simulink model "blockdemo"  (Simulink 6.3)
settings: Solver=FixedStepDiscrete  StartTime=0.0  StopTime=20  FixedStep=1  RelTol=1e-3
InitFcn:
  | %% DSPBuilder Start
  | alt_dspbuilder_update_model(bdroot)
  | %% DSPBuilder End
libraries: allblocks_alteradspbuilder2 x5
settings Model: Creator=cpurcell  LastModifiedBy=delphick
settings OptimizationCC: BlockReduction=off  BooleanDataType=off  InlineInvariantSignals=on
settings DebuggingCC: SolverPrmCheckMsg=none
settings HardwareCC: TargetUnknown=on

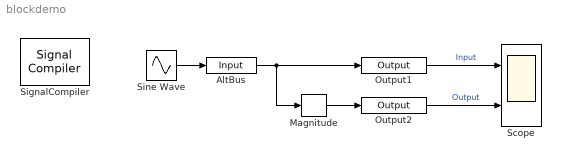
== system blockdemo ==
  AltBus : allblocks_alteradspbuilder2/Input  iofile=C:\workspace_clean\Documentation\DesignExamples\Tutorials\UnitBlocks\Arithmetic\Magnitude\tb_blockdemo\blockdemo_AltBus.salt  BusType=Signed Integer  bwl=5  bwr=4  SpecifyClock=off  PORTTYPE=Input
  Magnitude : allblocks_alteradspbuilder2/Magnitude
  Output1 : allblocks_alteradspbuilder2/Output  iofile=C:\workspace_clean\Documentation\DesignExamples\Tutorials\UnitBlocks\Arithmetic\Magnitude\tb_blockdemo\blockdemo_Output1.capture  BusType=Signed Integer  bwl=5  bwr=0  PORTTYPE=Output
  Output2 : allblocks_alteradspbuilder2/Output  iofile=C:\workspace_clean\Documentation\DesignExamples\Tutorials\UnitBlocks\Arithmetic\Magnitude\tb_blockdemo\blockdemo_Output2.capture  BusType=Signed Integer  bwl=5  bwr=0  PORTTYPE=Output
  Scope : Scope  NumInputPorts=2
      settings: YMin=-20~0  YMax=20~16
  SignalCompiler : allblocks_alteradspbuilder2/Signal Compiler  DeviceFamily=Stratix IV  DeviceName=AUTO  EnableSignalTap=off  SignalTapDepth=128  UseBoardBlock=off  StpUseDefaultClock=on  StpClock=clock
  Sine Wave : Sin  SineType=Sample based  Amplitude=15  Frequency=0.4  Phase=2  Samples=15  SampleTime=1  Offset=4
  wires:
  AltBus/1 -> Magnitude/1, Output1/1
  Sine Wave/1 -> AltBus/1
  Magnitude/1 -> Output2/1
  Output2/1 -> Scope/2  "Output"
  Output1/1 -> Scope/1  "Input"
